simulink model "SecRwLtStLgrstInwdOtwdIsPosChk"  (R2024b)
settings: Solver=FixedStepDiscrete  StartTime=0.0  StopTime=10.0  FixedStep=0.01  RelTol=1e-3
undefined symbols (not defined in the file or in its folder): KeSMSuSecRwStLegrestInOutPosDelta_Val, KeSMSuSecRwStLegrestInOutPosTolr_Val
libraries: StIsPosChkLib x12, simulink x7
(part 1 of 2)
settings Model: Creator=sn2xws  LastModifiedBy=sn55gm
settings Model: ModifiedHistory=|
  | 2023.8.1 V2.0.0 CR421790 增加模式21-26
  | 2023.9.14 V2.1.0 Bug 540886 修改模式判断到位的条件为10ms周期计算
  | 2024.5.8 V3.0.0 557 eze 模式变更
  | 2024.8.15 V3.0.1 智享模式需要计算目标位置，不能直接判断到位置，posalready赋值0
  | 2024.9.5 V3.0.2 增加Md56，注释不用的模式
  | 2024.12.17 V3.0.3 Md57 Md58 报失败问题
  | 25.7.1 V3.13.0 新增MD61 MD62
  | 2510.10V3.13.2 二排腿托都动完再停发目标位置
settings SolverCC: AlgebraicLoopSolver=TrustRegion
settings DataIOCC: SaveFormat=StructureWithTime  ReturnWorkspaceOutputs=off
settings OptimizationCC: DefaultParameterBehavior=Inlined  EnhancedBackFolding=on  PassReuseOutputArgsAs=Individual arguments  ZeroExternalMemoryAtStartup=off  ZeroInternalMemoryAtStartup=off  OptimizeBlockOrder=speed  DifferentSizesBufferReuse=on  OptimizationCustomize=off  EfficientTunableParamExpr=on
settings DebuggingCC: ParameterTunabilityLossMsg=error  UnconnectedInputMsg=warning  UnconnectedOutputMsg=warning  UnconnectedLineMsg=warning  ArithmeticOperatorsInVariantConditions=warning
settings ModelReferenceCC: EnableRefExpFcnMdlSchedulingChecks=on  ModelReferenceNumInstancesAllowed=Single
settings SFSimCC: MATLABDynamicMemAlloc=off  CustomCodeUndefinedFunction=UseInterfaceOnly
settings RTWCC: Description=AUTOSAR  SystemTargetFile=autosar.tlc  GenCodeOnly=on  TemplateMakefile=ert_default_tmf  GenerateReport=on  IncludeHyperlinkInReport=on  LaunchReport=on  DataTypeReplacement=CDataTypesFixedWidth  GenerateTraceInfo=on  GenerateTraceReport=on  GenerateTraceReportSl=on  GenerateTraceReportSf=on  GenerateTraceReportEml=on  GenerateCodeMetricsReport=on  GPUComputeCapability=3.5
settings CodeAppCC: ForceParamTrailComments=on  IgnoreCustomStorageClasses=off  OperatorAnnotations=on  SimulinkDataObjDesc=on  SFDataObjDesc=on  InsertBlockDesc=on
settings STFCustomTargetCC: TargetLangStandard=C99 (ISO)  MultiwordLength=256  ParMdlRefBuildCompliant=on  CompOptLevelCompliant=on  IncludeMdlTerminateFcn=off  CombineOutputUpdateFcns=on  SuppressErrorStatus=on  ERTCustomFileBanners=on  SupportNonFinite=off  SupportComplex=off  SupportContinuousTime=off  SupportNonInlinedSFcns=off  RemoveResetFunc=on  MATLABClassNameForMDSCustomization=Simulink.SoftwareTarget.ERTCustomization  AutosarCompliant=on  UseToolchainInfoCompliant=on  LookupTableObjectStructAxisOrder=2,1,3,4,...  LUTObjectStructOrderEvenSpacing=Size,Table,Breakpoints  SystemTargetFile=autosar.tlc
settings ERTTargetCC: TargetLangStandard=C99 (ISO)  ConcurrentExecutionCompliant=off  IncludeMdlTerminateFcn=off  SuppressErrorStatus=on  SupportNonFinite=off  SupportComplex=off  ModelStepFunctionPrototypeControlCompliant=off  CPPClassGenCompliant=off  AutosarCompliant=on  LookupTableObjectStructAxisOrder=2,1,3,4,...  LUTObjectStructOrderEvenSpacing=Size,Table,Breakpoints  ERTCustomFileTemplate=example_file_process.tlc  ERTFilePackagingFormat=Compact  BooleanTrueId=TRUE  BooleanFalseId=FALSE  DynamicArrayContainerType=coder::array

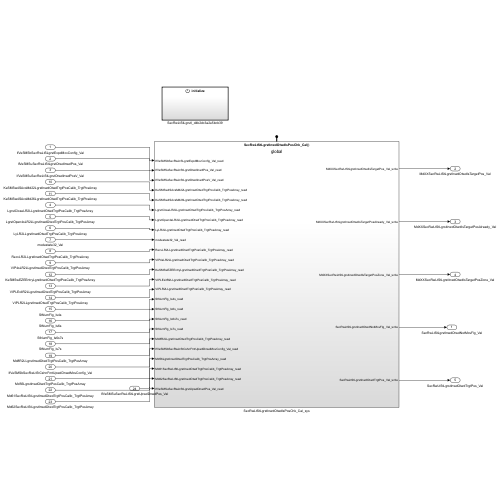
[thumbnail: Simulink's stored preview of the top-level diagram]
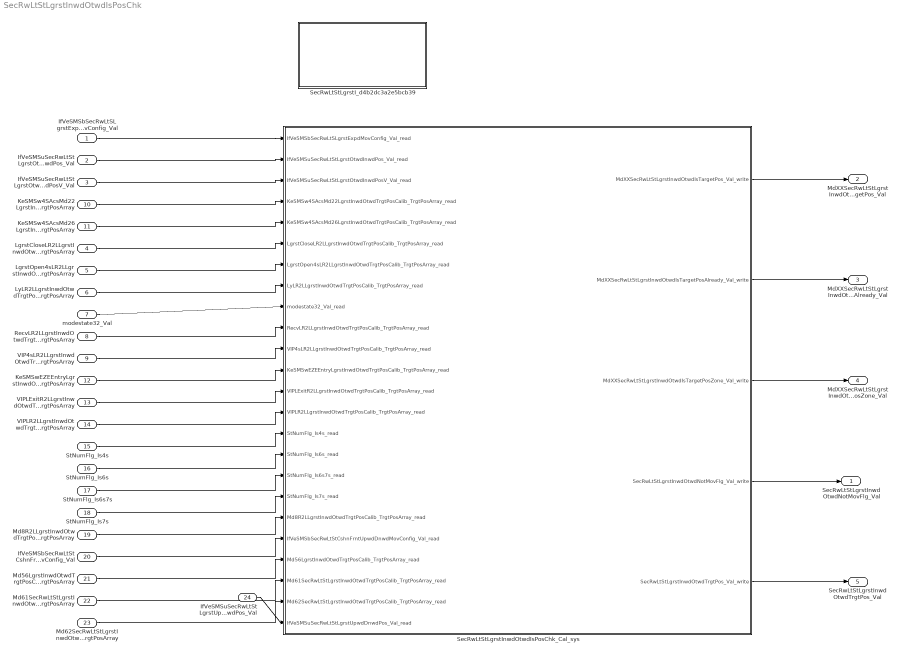
== system SecRwLtStLgrstInwdOtwdIsPosChk ==
  IfVeSMSbSecRwLtSLgrstExpdMovConfig_Val : Inport  OutDataTypeStr=boolean  PortDimensions=1
  IfVeSMSuSecRwLtStLgrstOtwdInwdPos_Val : Inport  Port=2  OutDataTypeStr=uint16  PortDimensions=1
  IfVeSMSuSecRwLtStLgrstOtwdInwdPosV_Val : Inport  Port=3  OutDataTypeStr=boolean  PortDimensions=1
  LgrstCloseLR2LLgrstInwdOtwdTrgtPosCalib_TrgtPosArray : Inport  Description=|  Port=4  OutDataTypeStr=uint16  PortDimensions=3
      | 0:Pos
      | 1:Max
      | 2:Min
  LgrstOpen4sLR2LLgrstInwdOtwdTrgtPosCalib_TrgtPosArray : Inport  Description=|  Port=5  OutDataTypeStr=uint16  PortDimensions=3
      | 0:Pos
      | 1:Max
      | 2:Min
  LyLR2LLgrstInwdOtwdTrgtPosCalib_TrgtPosArray : Inport  Description=|  Port=6  OutDataTypeStr=uint16  PortDimensions=3
      | 0:Pos
      | 1:Max
      | 2:Min
  modestate32_Val : Inport  Port=7  OutDataTypeStr=uint32  PortDimensions=1
  RecvLR2LLgrstInwdOtwdTrgtPosCalib_TrgtPosArray : Inport  Description=|  Port=8  OutDataTypeStr=uint16  PortDimensions=3
      | 0:Pos
      | 1:Max
      | 2:Min
  VIP4sLR2LLgrstInwdOtwdTrgtPosCalib_TrgtPosArray : Inport  Description=|  Port=9  OutDataTypeStr=uint16  PortDimensions=3
      | 0:Pos
      | 1:Max
      | 2:Min
  KeSMSw4SAcsMd22LgrstInwdOtwdTrgtPosCalib_TrgtPosArray : Inport  Description=|  Port=10  OutDataTypeStr=uint16  PortDimensions=3
      | 0:Pos
      | 1:Max
      | 2:Min
  KeSMSw4SAcsMd26LgrstInwdOtwdTrgtPosCalib_TrgtPosArray : Inport  Description=|  Port=11  OutDataTypeStr=uint16  PortDimensions=3
      | 0:Pos
      | 1:Max
      | 2:Min
  KeSMSwEZEEntryLgrstInwdOtwdTrgtPosCalib_TrgtPosArray : Inport  Description=|  Port=12  OutDataTypeStr=uint16  PortDimensions=3
      | 0:Pos
      | 1:Max
      | 2:Min
  VIPLExitR2LLgrstInwdOtwdTrgtPosCalib_TrgtPosArray : Inport  Description=|  Port=13  OutDataTypeStr=uint16  PortDimensions=3
      | 0:Pos
      | 1:Max
      | 2:Min
  VIPLR2LLgrstInwdOtwdTrgtPosCalib_TrgtPosArray : Inport  Description=|  Port=14  OutDataTypeStr=uint16  PortDimensions=3
      | 0:Pos
      | 1:Max
      | 2:Min
  StNumFlg_Is4s : Inport  Port=15  OutDataTypeStr=boolean  PortDimensions=1
  StNumFlg_Is6s : Inport  Port=16  OutDataTypeStr=boolean  PortDimensions=1
  StNumFlg_Is6s7s : Inport  Port=17  OutDataTypeStr=boolean  PortDimensions=1
  StNumFlg_Is7s : Inport  Port=18  OutDataTypeStr=boolean  PortDimensions=1
  Md8R2LLgrstInwdOtwdTrgtPosCalib_TrgtPosArray : Inport  Description=|  Port=19  OutDataTypeStr=uint16  PortDimensions=3
      | 0:Pos
      | 1:Max
      | 2:Min
  IfVeSMSbSecRwLtStCshnFrntUpwdDnwdMovConfig_Val : Inport  Port=20  OutDataTypeStr=boolean  PortDimensions=1
  Md56LgrstInwdOtwdTrgtPosCalib_TrgtPosArray : Inport  Description=|  Port=21  OutDataTypeStr=uint16  PortDimensions=3
      | 0:Pos
      | 1:Max
      | 2:Min
  Md61SecRwLtStLgrstInwdOtwdTrgtPosCalib_TrgtPosArray : Inport  Description=|  Port=22  OutDataTypeStr=uint16  PortDimensions=3
      | 0:Pos
      | 1:Max
      | 2:Min
  Md62SecRwLtStLgrstInwdOtwdTrgtPosCalib_TrgtPosArray : Inport  Description=|  Port=23  OutDataTypeStr=uint16  PortDimensions=3
      | 0:Pos
      | 1:Max
      | 2:Min
  IfVeSMSuSecRwLtStLgrstUpwdDnwdPos_Val : Inport  Port=24  OutDataTypeStr=uint16  PortDimensions=1
  SecRwLtStLgrstI_d4b2dc3a2e5bcb39 : Subsystem
  SecRwLtStLgrstInwdOtwdIsPosChk_Cal_sys : Subsystem
  SecRwLtStLgrstInwdOtwdNotMovFlg_Val : Outport  OutDataTypeStr=boolean  PortDimensions=1  VectorParamsAs1DForOutWhenUnconnected=off
  MdXXSecRwLtStLgrstInwdOtwdIsTargetPos_Val : Outport  Port=2  OutDataTypeStr=uint32  PortDimensions=1  VectorParamsAs1DForOutWhenUnconnected=off
  MdXXSecRwLtStLgrstInwdOtwdIsTargetPosAlready_Val : Outport  Port=3  OutDataTypeStr=uint32  PortDimensions=1  VectorParamsAs1DForOutWhenUnconnected=off
  MdXXSecRwLtStLgrstInwdOtwdIsTargetPosZone_Val : Outport  Port=4  OutDataTypeStr=uint32  PortDimensions=1  VectorParamsAs1DForOutWhenUnconnected=off
  SecRwLtStLgrstInwdOtwdTrgtPos_Val : Outport  Port=5  OutDataTypeStr=uint16  PortDimensions=1  VectorParamsAs1DForOutWhenUnconnected=off
  wires:
  IfVeSMSbSecRwLtSLgrstExpdMovConfig_Val/1 -> SecRwLtStLgrstInwdOtwdIsPosChk_Cal_sys/1(IfVeSMSbSecRwLtSLgrstExpdMovConfig_Val_read)
  IfVeSMSuSecRwLtStLgrstOtwdInwdPos_Val/1 -> SecRwLtStLgrstInwdOtwdIsPosChk_Cal_sys/2(IfVeSMSuSecRwLtStLgrstOtwdInwdPos_Val_read)
  IfVeSMSuSecRwLtStLgrstOtwdInwdPosV_Val/1 -> SecRwLtStLgrstInwdOtwdIsPosChk_Cal_sys/3(IfVeSMSuSecRwLtStLgrstOtwdInwdPosV_Val_read)
  LgrstCloseLR2LLgrstInwdOtwdTrgtPosCalib_TrgtPosArray/1 -> SecRwLtStLgrstInwdOtwdIsPosChk_Cal_sys/6(LgrstCloseLR2LLgrstInwdOtwdTrgtPosCalib_TrgtPosArray_read)
  LgrstOpen4sLR2LLgrstInwdOtwdTrgtPosCalib_TrgtPosArray/1 -> SecRwLtStLgrstInwdOtwdIsPosChk_Cal_sys/7(LgrstOpen4sLR2LLgrstInwdOtwdTrgtPosCalib_TrgtPosArray_read)
  LyLR2LLgrstInwdOtwdTrgtPosCalib_TrgtPosArray/1 -> SecRwLtStLgrstInwdOtwdIsPosChk_Cal_sys/8(LyLR2LLgrstInwdOtwdTrgtPosCalib_TrgtPosArray_read)
  modestate32_Val/1 -> SecRwLtStLgrstInwdOtwdIsPosChk_Cal_sys/9(modestate32_Val_read)
  RecvLR2LLgrstInwdOtwdTrgtPosCalib_TrgtPosArray/1 -> SecRwLtStLgrstInwdOtwdIsPosChk_Cal_sys/10(RecvLR2LLgrstInwdOtwdTrgtPosCalib_TrgtPosArray_read)
  VIP4sLR2LLgrstInwdOtwdTrgtPosCalib_TrgtPosArray/1 -> SecRwLtStLgrstInwdOtwdIsPosChk_Cal_sys/11(VIP4sLR2LLgrstInwdOtwdTrgtPosCalib_TrgtPosArray_read)
  SecRwLtStLgrstInwdOtwdIsPosChk_Cal_sys/1(MdXXSecRwLtStLgrstInwdOtwdIsTargetPos_Val_write) -> MdXXSecRwLtStLgrstInwdOtwdIsTargetPos_Val/1
  SecRwLtStLgrstInwdOtwdIsPosChk_Cal_sys/2(MdXXSecRwLtStLgrstInwdOtwdIsTargetPosAlready_Val_write) -> MdXXSecRwLtStLgrstInwdOtwdIsTargetPosAlready_Val/1
  SecRwLtStLgrstInwdOtwdIsPosChk_Cal_sys/3(MdXXSecRwLtStLgrstInwdOtwdIsTargetPosZone_Val_write) -> MdXXSecRwLtStLgrstInwdOtwdIsTargetPosZone_Val/1
  SecRwLtStLgrstInwdOtwdIsPosChk_Cal_sys/4(SecRwLtStLgrstInwdOtwdNotMovFlg_Val_write) -> SecRwLtStLgrstInwdOtwdNotMovFlg_Val/1
  SecRwLtStLgrstInwdOtwdIsPosChk_Cal_sys/5(SecRwLtStLgrstInwdOtwdTrgtPos_Val_write) -> SecRwLtStLgrstInwdOtwdTrgtPos_Val/1
  KeSMSw4SAcsMd22LgrstInwdOtwdTrgtPosCalib_TrgtPosArray/1 -> SecRwLtStLgrstInwdOtwdIsPosChk_Cal_sys/4(KeSMSw4SAcsMd22LgrstInwdOtwdTrgtPosCalib_TrgtPosArray_read)
  KeSMSw4SAcsMd26LgrstInwdOtwdTrgtPosCalib_TrgtPosArray/1 -> SecRwLtStLgrstInwdOtwdIsPosChk_Cal_sys/5(KeSMSw4SAcsMd26LgrstInwdOtwdTrgtPosCalib_TrgtPosArray_read)
  KeSMSwEZEEntryLgrstInwdOtwdTrgtPosCalib_TrgtPosArray/1 -> SecRwLtStLgrstInwdOtwdIsPosChk_Cal_sys/12(KeSMSwEZEEntryLgrstInwdOtwdTrgtPosCalib_TrgtPosArray_read)
  VIPLExitR2LLgrstInwdOtwdTrgtPosCalib_TrgtPosArray/1 -> SecRwLtStLgrstInwdOtwdIsPosChk_Cal_sys/13(VIPLExitR2LLgrstInwdOtwdTrgtPosCalib_TrgtPosArray_read)
  VIPLR2LLgrstInwdOtwdTrgtPosCalib_TrgtPosArray/1 -> SecRwLtStLgrstInwdOtwdIsPosChk_Cal_sys/14(VIPLR2LLgrstInwdOtwdTrgtPosCalib_TrgtPosArray_read)
  StNumFlg_Is4s/1 -> SecRwLtStLgrstInwdOtwdIsPosChk_Cal_sys/15(StNumFlg_Is4s_read)
  StNumFlg_Is6s/1 -> SecRwLtStLgrstInwdOtwdIsPosChk_Cal_sys/16(StNumFlg_Is6s_read)
  StNumFlg_Is6s7s/1 -> SecRwLtStLgrstInwdOtwdIsPosChk_Cal_sys/17(StNumFlg_Is6s7s_read)
  StNumFlg_Is7s/1 -> SecRwLtStLgrstInwdOtwdIsPosChk_Cal_sys/18(StNumFlg_Is7s_read)
  Md8R2LLgrstInwdOtwdTrgtPosCalib_TrgtPosArray/1 -> SecRwLtStLgrstInwdOtwdIsPosChk_Cal_sys/19(Md8R2LLgrstInwdOtwdTrgtPosCalib_TrgtPosArray_read)
  IfVeSMSbSecRwLtStCshnFrntUpwdDnwdMovConfig_Val/1 -> SecRwLtStLgrstInwdOtwdIsPosChk_Cal_sys/20(IfVeSMSbSecRwLtStCshnFrntUpwdDnwdMovConfig_Val_read)
  Md56LgrstInwdOtwdTrgtPosCalib_TrgtPosArray/1 -> SecRwLtStLgrstInwdOtwdIsPosChk_Cal_sys/21(Md56LgrstInwdOtwdTrgtPosCalib_TrgtPosArray_read)
  Md61SecRwLtStLgrstInwdOtwdTrgtPosCalib_TrgtPosArray/1 -> SecRwLtStLgrstInwdOtwdIsPosChk_Cal_sys/22(Md61SecRwLtStLgrstInwdOtwdTrgtPosCalib_TrgtPosArray_read)
  Md62SecRwLtStLgrstInwdOtwdTrgtPosCalib_TrgtPosArray/1 -> SecRwLtStLgrstInwdOtwdIsPosChk_Cal_sys/23(Md62SecRwLtStLgrstInwdOtwdTrgtPosCalib_TrgtPosArray_read)
  IfVeSMSuSecRwLtStLgrstUpwdDnwdPos_Val/1 -> SecRwLtStLgrstInwdOtwdIsPosChk_Cal_sys/24(IfVeSMSuSecRwLtStLgrstUpwdDnwdPos_Val_read)

== system SecRwLtStLgrstInwdOtwdIsPosChk/SecRwLtStLgrstI_d4b2dc3a2e5bcb39 ==
  note: Added blocks
  note: Added blocks
  Event Listener : EventListener  EventName=reset
  PA_KeSMSuSecRwStLegrestInOutPosDelta_Val : Constant  Value=KeSMSuSecRwStLegrestInOutPosDelta_Val
  PA_KeSMSuSecRwStLegrestInOutPosTolr_Val : Constant  Value=KeSMSuSecRwStLegrestInOutPosTolr_Val
  Terminator_1 : Terminator
  Terminator_2 : Terminator
  wires:
  PA_KeSMSuSecRwStLegrestInOutPosDelta_Val/1 -> Terminator_1/1
  PA_KeSMSuSecRwStLegrestInOutPosTolr_Val/1 -> Terminator_2/1

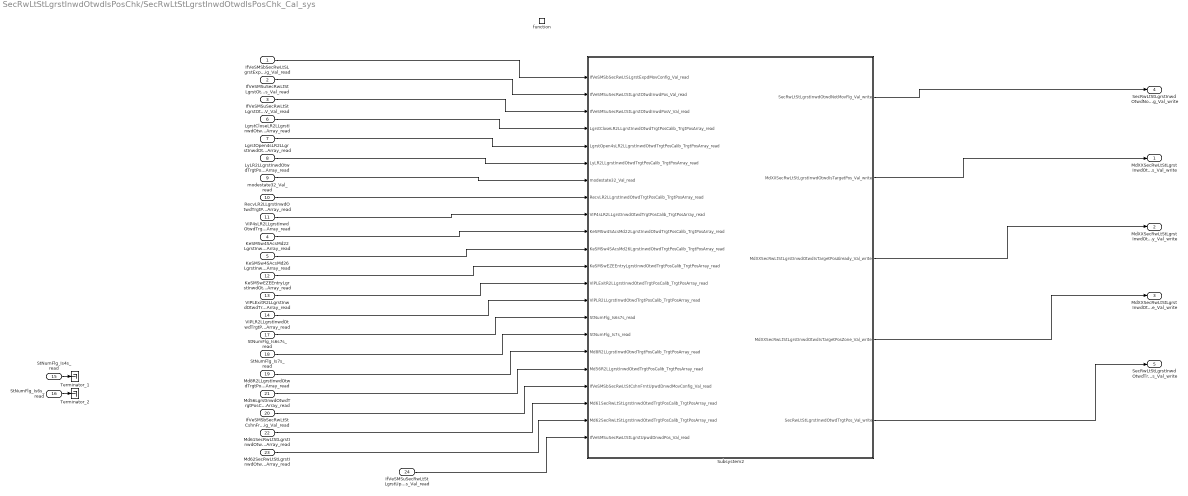
== system SecRwLtStLgrstInwdOtwdIsPosChk/SecRwLtStLgrstInwdOtwdIsPosChk_Cal_sys ==
  IfVeSMSbSecRwLtSLgrstExpdMovConfig_Val_read : Inport
  IfVeSMSuSecRwLtStLgrstOtwdInwdPos_Val_read : Inport  Port=2
  IfVeSMSuSecRwLtStLgrstOtwdInwdPosV_Val_read : Inport  Port=3
  KeSMSw4SAcsMd22LgrstInwdOtwdTrgtPosCalib_TrgtPosArray_read : Inport  Port=4
  KeSMSw4SAcsMd26LgrstInwdOtwdTrgtPosCalib_TrgtPosArray_read : Inport  Port=5
  LgrstCloseLR2LLgrstInwdOtwdTrgtPosCalib_TrgtPosArray_read : Inport  Port=6
  LgrstOpen4sLR2LLgrstInwdOtwdTrgtPosCalib_TrgtPosArray_read : Inport  Port=7
  LyLR2LLgrstInwdOtwdTrgtPosCalib_TrgtPosArray_read : Inport  Port=8
  modestate32_Val_read : Inport  Port=9
  RecvLR2LLgrstInwdOtwdTrgtPosCalib_TrgtPosArray_read : Inport  Port=10
  VIP4sLR2LLgrstInwdOtwdTrgtPosCalib_TrgtPosArray_read : Inport  Port=11
  KeSMSwEZEEntryLgrstInwdOtwdTrgtPosCalib_TrgtPosArray_read : Inport  Port=12
  VIPLExitR2LLgrstInwdOtwdTrgtPosCalib_TrgtPosArray_read : Inport  Port=13
  VIPLR2LLgrstInwdOtwdTrgtPosCalib_TrgtPosArray_read : Inport  Port=14
  StNumFlg_Is4s_read : Inport  Port=15
  StNumFlg_Is6s_read : Inport  Port=16
  StNumFlg_Is6s7s_read : Inport  Port=17
  StNumFlg_Is7s_read : Inport  Port=18
  Md8R2LLgrstInwdOtwdTrgtPosCalib_TrgtPosArray_read : Inport  Port=19
  IfVeSMSbSecRwLtStCshnFrntUpwdDnwdMovConfig_Val_read : Inport  Port=20
  Md56LgrstInwdOtwdTrgtPosCalib_TrgtPosArray_read : Inport  Port=21
  Md61SecRwLtStLgrstInwdOtwdTrgtPosCalib_TrgtPosArray_read : Inport  Port=22
  Md62SecRwLtStLgrstInwdOtwdTrgtPosCalib_TrgtPosArray_read : Inport  Port=23
  IfVeSMSuSecRwLtStLgrstUpwdDnwdPos_Val_read : Inport  Port=24
  function : TriggerPort  TriggerType=function-call  IsSimulinkFunction=on  FunctionName=SecRwLtStLgrstInwdOtwdIsPosChk_Cal  VariantControl=(inherit)
  Subsystem2 : Subsystem
  Terminator_1 : Terminator
  Terminator_2 : Terminator
  MdXXSecRwLtStLgrstInwdOtwdIsTargetPos_Val_write : Outport  VectorParamsAs1DForOutWhenUnconnected=off
      settings: EnsureOutportIsVirtual=on
  MdXXSecRwLtStLgrstInwdOtwdIsTargetPosAlready_Val_write : Outport  Port=2  VectorParamsAs1DForOutWhenUnconnected=off
      settings: EnsureOutportIsVirtual=on
  MdXXSecRwLtStLgrstInwdOtwdIsTargetPosZone_Val_write : Outport  Port=3  VectorParamsAs1DForOutWhenUnconnected=off
      settings: EnsureOutportIsVirtual=on
  SecRwLtStLgrstInwdOtwdNotMovFlg_Val_write : Outport  Port=4  VectorParamsAs1DForOutWhenUnconnected=off
      settings: EnsureOutportIsVirtual=on
  SecRwLtStLgrstInwdOtwdTrgtPos_Val_write : Outport  Port=5  VectorParamsAs1DForOutWhenUnconnected=off
      settings: EnsureOutportIsVirtual=on
  wires:
  LgrstCloseLR2LLgrstInwdOtwdTrgtPosCalib_TrgtPosArray_read/1 -> Subsystem2/4(LgrstCloseLR2LLgrstInwdOtwdTrgtPosCalib_TrgtPosArray_read)
  IfVeSMSuSecRwLtStLgrstOtwdInwdPos_Val_read/1 -> Subsystem2/2(IfVeSMSuSecRwLtStLgrstOtwdInwdPos_Val_read)
  IfVeSMSuSecRwLtStLgrstOtwdInwdPosV_Val_read/1 -> Subsystem2/3(IfVeSMSuSecRwLtStLgrstOtwdInwdPosV_Val_read)
  LgrstOpen4sLR2LLgrstInwdOtwdTrgtPosCalib_TrgtPosArray_read/1 -> Subsystem2/5(LgrstOpen4sLR2LLgrstInwdOtwdTrgtPosCalib_TrgtPosArray_read)
  IfVeSMSbSecRwLtSLgrstExpdMovConfig_Val_read/1 -> Subsystem2/1(IfVeSMSbSecRwLtSLgrstExpdMovConfig_Val_read)
  LyLR2LLgrstInwdOtwdTrgtPosCalib_TrgtPosArray_read/1 -> Subsystem2/6(LyLR2LLgrstInwdOtwdTrgtPosCalib_TrgtPosArray_read)
  modestate32_Val_read/1 -> Subsystem2/7(modestate32_Val_read)
  RecvLR2LLgrstInwdOtwdTrgtPosCalib_TrgtPosArray_read/1 -> Subsystem2/8(RecvLR2LLgrstInwdOtwdTrgtPosCalib_TrgtPosArray_read)
  VIP4sLR2LLgrstInwdOtwdTrgtPosCalib_TrgtPosArray_read/1 -> Subsystem2/9(VIP4sLR2LLgrstInwdOtwdTrgtPosCalib_TrgtPosArray_read)
  KeSMSw4SAcsMd22LgrstInwdOtwdTrgtPosCalib_TrgtPosArray_read/1 -> Subsystem2/10(KeSMSw4SAcsMd22LgrstInwdOtwdTrgtPosCalib_TrgtPosArray_read)
  KeSMSw4SAcsMd26LgrstInwdOtwdTrgtPosCalib_TrgtPosArray_read/1 -> Subsystem2/11(KeSMSw4SAcsMd26LgrstInwdOtwdTrgtPosCalib_TrgtPosArray_read)
  Subsystem2/1(SecRwLtStLgrstInwdOtwdNotMovFlg_Val_write) -> SecRwLtStLgrstInwdOtwdNotMovFlg_Val_write/1
  Subsystem2/2(MdXXSecRwLtStLgrstInwdOtwdIsTargetPos_Val_write) -> MdXXSecRwLtStLgrstInwdOtwdIsTargetPos_Val_write/1
  Subsystem2/3(MdXXSecRwLtStLgrstInwdOtwdIsTargetPosAlready_Val_write) -> MdXXSecRwLtStLgrstInwdOtwdIsTargetPosAlready_Val_write/1
  Subsystem2/4(MdXXSecRwLtStLgrstInwdOtwdIsTargetPosZone_Val_write) -> MdXXSecRwLtStLgrstInwdOtwdIsTargetPosZone_Val_write/1
  Subsystem2/5(SecRwLtStLgrstInwdOtwdTrgtPos_Val_write) -> SecRwLtStLgrstInwdOtwdTrgtPos_Val_write/1
  KeSMSwEZEEntryLgrstInwdOtwdTrgtPosCalib_TrgtPosArray_read/1 -> Subsystem2/12(KeSMSwEZEEntryLgrstInwdOtwdTrgtPosCalib_TrgtPosArray_read)
  VIPLExitR2LLgrstInwdOtwdTrgtPosCalib_TrgtPosArray_read/1 -> Subsystem2/13(VIPLExitR2LLgrstInwdOtwdTrgtPosCalib_TrgtPosArray_read)
  VIPLR2LLgrstInwdOtwdTrgtPosCalib_TrgtPosArray_read/1 -> Subsystem2/14(VIPLR2LLgrstInwdOtwdTrgtPosCalib_TrgtPosArray_read)
  StNumFlg_Is4s_read/1 -> Terminator_1/1
  StNumFlg_Is6s_read/1 -> Terminator_2/1
  StNumFlg_Is6s7s_read/1 -> Subsystem2/15(StNumFlg_Is6s7s_read)
  StNumFlg_Is7s_read/1 -> Subsystem2/16(StNumFlg_Is7s_read)
  Md8R2LLgrstInwdOtwdTrgtPosCalib_TrgtPosArray_read/1 -> Subsystem2/17(Md8R2LLgrstInwdOtwdTrgtPosCalib_TrgtPosArray_read)
  Md56LgrstInwdOtwdTrgtPosCalib_TrgtPosArray_read/1 -> Subsystem2/18(Md56R2LLgrstInwdOtwdTrgtPosCalib_TrgtPosArray_read)
  IfVeSMSbSecRwLtStCshnFrntUpwdDnwdMovConfig_Val_read/1 -> Subsystem2/19(IfVeSMSbSecRwLtStCshnFrntUpwdDnwdMovConfig_Val_read)
  Md61SecRwLtStLgrstInwdOtwdTrgtPosCalib_TrgtPosArray_read/1 -> Subsystem2/20(Md61SecRwLtStLgrstInwdOtwdTrgtPosCalib_TrgtPosArray_read)
  Md62SecRwLtStLgrstInwdOtwdTrgtPosCalib_TrgtPosArray_read/1 -> Subsystem2/21(Md62SecRwLtStLgrstInwdOtwdTrgtPosCalib_TrgtPosArray_read)
  IfVeSMSuSecRwLtStLgrstUpwdDnwdPos_Val_read/1 -> Subsystem2/22(IfVeSMSuSecRwLtStLgrstUpwdDnwdPos_Val_read)

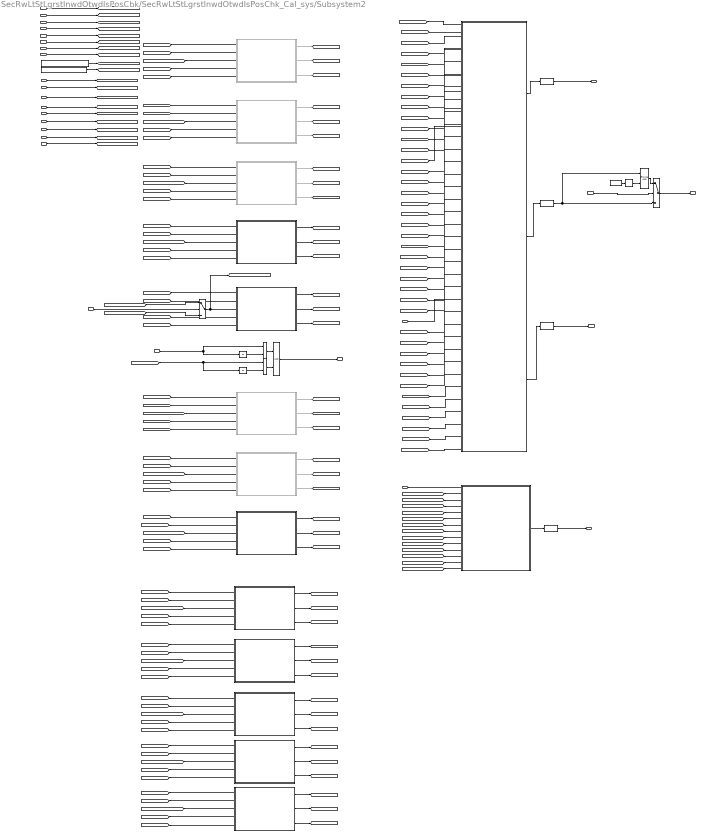
== system SecRwLtStLgrstInwdOtwdIsPosChk/SecRwLtStLgrstInwdOtwdIsPosChk_Cal_sys/Subsystem2 ==
  note: 2023.9.14 V2.1.0 Bug 540886 修改模式判断到位的条件为10ms周期计算
  note: 2023.8.1 V2.0.0 CR421790 增加模式21-26
  IfVeSMSbSecRwLtSLgrstExpdMovConfig_Val_read : Inport
  IfVeSMSuSecRwLtStLgrstOtwdInwdPos_Val_read : Inport  Port=2
  IfVeSMSuSecRwLtStLgrstOtwdInwdPosV_Val_read : Inport  Port=3
  LgrstCloseLR2LLgrstInwdOtwdTrgtPosCalib_TrgtPosArray_read : Inport  Port=4
  LgrstOpen4sLR2LLgrstInwdOtwdTrgtPosCalib_TrgtPosArray_read : Inport  Port=5
  LyLR2LLgrstInwdOtwdTrgtPosCalib_TrgtPosArray_read : Inport  Port=6
  modestate32_Val_read : Inport  Port=7
  RecvLR2LLgrstInwdOtwdTrgtPosCalib_TrgtPosArray_read : Inport  Port=8
  VIP4sLR2LLgrstInwdOtwdTrgtPosCalib_TrgtPosArray_read : Inport  Port=9
  KeSMSw4SAcsMd22LgrstInwdOtwdTrgtPosCalib_TrgtPosArray_read : Inport  Port=10
  KeSMSw4SAcsMd26LgrstInwdOtwdTrgtPosCalib_TrgtPosArray_read : Inport  Port=11
  KeSMSwEZEEntryLgrstInwdOtwdTrgtPosCalib_TrgtPosArray_read : Inport  Port=12
  VIPLExitR2LLgrstInwdOtwdTrgtPosCalib_TrgtPosArray_read : Inport  Port=13
  VIPLR2LLgrstInwdOtwdTrgtPosCalib_TrgtPosArray_read : Inport  Port=14
  StNumFlg_Is6s7s_read : Inport  Port=15
  StNumFlg_Is7s_read : Inport  Port=16
  Md8R2LLgrstInwdOtwdTrgtPosCalib_TrgtPosArray_read : Inport  Port=17
  Md56R2LLgrstInwdOtwdTrgtPosCalib_TrgtPosArray_read : Inport  Port=18
  IfVeSMSbSecRwLtStCshnFrntUpwdDnwdMovConfig_Val_read : Inport  Port=19
  Md61SecRwLtStLgrstInwdOtwdTrgtPosCalib_TrgtPosArray_read : Inport  Port=20
  Md62SecRwLtStLgrstInwdOtwdTrgtPosCalib_TrgtPosArray_read : Inport  Port=21
  IfVeSMSuSecRwLtStLgrstUpwdDnwdPos_Val_read : Inport  Port=22
  Bitwise Operator : simulink/Logic and Bit Operations/Bitwise Operator  logicop=AND  UseBitMask=off  NumInputPorts=2  BitMask=bin2dec('11011001')  BitMaskRealWorld=Stored Integer
  Bitwise Operator1 : simulink/Logic and Bit Operations/Bitwise Operator  logicop=NOT  UseBitMask=off  BitMask=bin2dec('11011001')  BitMaskRealWorld=Stored Integer
  Constant : Constant  Value=512  OutDataTypeStr=uint32
  Data Type Conversion{,1..3} (4 alike) : DataTypeConversion  SaturateOnIntegerOverflow=off  RndMeth=Floor
  Logical Operator3 : Logic  AllPortsSameDT=off  OutDataTypeStr=boolean
  PA_KeSMSuSecRwStLegrestInOutPosDelta_Val : Constant  Value=KeSMSuSecRwStLegrestInOutPosDelta_Val
  PA_KeSMSuSecRwStLegrestInOutPosTolr_Val : Constant  Value=KeSMSuSecRwStLegrestInOutPosTolr_Val
  Relational Operator2 : RelationalOperator  Operator===  OutDataTypeStr=boolean  RndMeth=Simplest  InputSameDT=off
  Relational Operator3 : RelationalOperator  Operator===  OutDataTypeStr=boolean  RndMeth=Simplest  InputSameDT=off
  Subsystem : Subsystem
  Subsystem1 : Subsystem
  Subsystem10 : Subsystem
  Subsystem11 : Subsystem
  Subsystem12 : Subsystem
  Subsystem13 : Subsystem
  Subsystem14 : Subsystem
  Subsystem2 : Subsystem  Commented=on
  Subsystem3 : Subsystem  Commented=on
  Subsystem4 : Subsystem  Commented=on
  Subsystem5 : Subsystem
  Subsystem6 : Subsystem
  Subsystem7 : Subsystem  Commented=on
  Subsystem8 : Subsystem  Commented=on
  Subsystem9 : Subsystem
  Switch : Switch  Criteria=u2 > Threshold  SaturateOnIntegerOverflow=off  InputSameDT=off
  Switch1 : Switch  Criteria=u2 > Threshold  SaturateOnIntegerOverflow=off  InputSameDT=off
  Unit Delay2 : UnitDelay  SampleTime=-1  HasFrameUpgradeWarning=on
  Unit Delay3 : UnitDelay  SampleTime=-1  HasFrameUpgradeWarning=on
  SecRwLtStLgrstInwdOtwdNotMovFlg_Val_write : Outport  VectorParamsAs1DForOutWhenUnconnected=off
      settings: EnsureOutportIsVirtual=on
  MdXXSecRwLtStLgrstInwdOtwdIsTargetPos_Val_write : Outport  Port=2  VectorParamsAs1DForOutWhenUnconnected=off
      settings: EnsureOutportIsVirtual=on
  MdXXSecRwLtStLgrstInwdOtwdIsTargetPosAlready_Val_write : Outport  Port=3  VectorParamsAs1DForOutWhenUnconnected=off
      settings: EnsureOutportIsVirtual=on
  MdXXSecRwLtStLgrstInwdOtwdIsTargetPosZone_Val_write : Outport  Port=4  VectorParamsAs1DForOutWhenUnconnected=off
      settings: EnsureOutportIsVirtual=on
  SecRwLtStLgrstInwdOtwdTrgtPos_Val_write : Outport  Port=5  VectorParamsAs1DForOutWhenUnconnected=off
      settings: EnsureOutportIsVirtual=on
  wires:
  [PosTolr] -> Subsystem5/5(Tolr)
  PA_KeSMSuSecRwStLegrestInOutPosTolr_Val/1 -> [PosTolr]
  [PosTolr] -> Subsystem6/5(Tolr)
  LgrstCloseLR2LLgrstInwdOtwdTrgtPosCalib_TrgtPosArray_read/1 -> [LgrstCloseLCalib]
  Subsystem1/3(IsTargetPosZone) -> Data Type Conversion3/1
  [PosTolr] -> Subsystem4/5(Tolr)
  [LgrstOpenLIsTargetPosAlready] -> ?
  [LgrstOpenLCalib] -> Subsystem/2(LgrstOpenLCalib)
  [PosTolr] -> Subsystem3/5(Tolr)
  Subsystem1/1(IsTargetPos) -> Data Type Conversion1/1
  IfVeSMSuSecRwLtStLgrstOtwdInwdPosV_Val_read/1 -> [PosV]
  [LgrstOpenLIsTargetPos] -> ?
  VIP4sLR2LLgrstInwdOtwdTrgtPosCalib_TrgtPosArray_read/1 -> [VIPL4sCalib]
  Subsystem4/2(IsPosZone) -> [LyLIsTargetPosZone]
  [VIPLIsTargetPosAlready] -> Subsystem1/7(VIPLIsTargetPosAlready)
  [VIPLCalib] -> Subsystem/6(VIPLCalib)
  [PosDelta] -> Subsystem3/4(Delta)
  [Pos] -> Subsystem3/2(Pos)
  Subsystem2/2(IsPosZone) -> [LgrstOpenLIsTargetPosZone]
  IfVeSMSbSecRwLtSLgrstExpdMovConfig_Val_read/1 -> [MovConfig]
  PA_KeSMSuSecRwStLegrestInOutPosDelta_Val/1 -> [PosDelta]
  [PosDelta] -> Subsystem6/4(Delta)
  LyLR2LLgrstInwdOtwdTrgtPosCalib_TrgtPosArray_read/1 -> [LyLCalib]
  LgrstOpen4sLR2LLgrstInwdOtwdTrgtPosCalib_TrgtPosArray_read/1 -> [LgrstOpenLCalib]
  [LgrstOpenLIsTargetPosZone] -> ?
  [LgrstCloseLIsTargetPosZone] -> Subsystem1/8(LgrstCloseLIsTargetPosZone)
  [VIPLIsTargetPosZone] -> Subsystem1/10(VIPLIsTargetPosZone)
  [PosDelta] -> Subsystem4/4(Delta)
  Subsystem5/2(IsPosZone) -> [RecvLIsTargetPosZone]
  [RecvLCalib] -> Subsystem/5(RecvLCalib)
  [RecvLIsTargetPosAlready] -> Subsystem1/6(RecvLIsTargetPosAlready)
  [RecvLCalib] -> Subsystem5/3(CalibArray)
  [LyLIsTargetPos] -> ?
  [LyLIsTargetPosAlready] -> ?
  [RecvLIsTargetPos] -> Subsystem1/3(RecvLIsTargetPos)
  Subsystem1/2(IsTargetPosAlready) -> Data Type Conversion2/1
  [LgrstCloseLIsTargetPosAlready] -> Subsystem1/5(LgrstCloseLIsTargetPosAlready)
  [PosDelta] -> Subsystem5/4(Delta)
  [VIPLIsTargetPos] -> Subsystem1/4(VIPLIsTargetPos)
  Subsystem5/1(IsPos) -> [RecvLIsTargetPos]
  Subsystem6/2(IsPosZone) -> [VIPLIsTargetPosZone]
  [LyLCalib] -> Subsystem4/3(CalibArray)
  [PosV] -> Subsystem2/1(PosV)
  IfVeSMSuSecRwLtStLgrstOtwdInwdPos_Val_read/1 -> [Pos]
  Data Type Conversion3/1 -> MdXXSecRwLtStLgrstInwdOtwdIsTargetPosZone_Val_write/1
  Subsystem5/3(IsPosAlready) -> [RecvLIsTargetPosAlready]
  [LyLCalib] -> Subsystem/4(LyLCalib)
  [PosV] -> Subsystem5/1(PosV)
  [PosV] -> Subsystem4/1(PosV)
  [LgrstCloseLIsTargetPos] -> Subsystem1/2(LgrstCloseLIsTargetPos)
  Subsystem/1(TrgtPos) -> Data Type Conversion/1
  [Pos] -> Subsystem6/2(Pos)
  Subsystem3/2(IsPosZone) -> [LgrstCloseLIsTargetPosZone]
  [RecvLIsTargetPosZone] -> Subsystem1/9(RecvLIsTargetPosZone)
  [Pos] -> Subsystem2/2(Pos)
  RecvLR2LLgrstInwdOtwdTrgtPosCalib_TrgtPosArray_read/1 -> [RecvLCalib]
  [Pos] -> Subsystem5/2(Pos)
  [LyLIsTargetPosZone] -> ?
  Subsystem3/1(IsPos) -> [LgrstCloseLIsTargetPos]
  Subsystem4/3(IsPosAlready) -> [LyLIsTargetPosAlready]
  [PosV] -> Subsystem3/1(PosV)
  [LgrstCloseLCalib] -> Subsystem/3(LgrstCloseLCalib)
  [MovConfig] -> Subsystem1/1(MovConfig)
  [PosTolr] -> Subsystem2/5(Tolr)
  Data Type Conversion/1 -> SecRwLtStLgrstInwdOtwdTrgtPos_Val_write/1
  [PosDelta] -> Subsystem2/4(Delta)
  Subsystem6/1(IsPos) -> [VIPLIsTargetPos]
  [Pos] -> Subsystem4/2(Pos)
  Subsystem3/3(IsPosAlready) -> [LgrstCloseLIsTargetPosAlready]
  Subsystem2/3(IsPosAlready) -> [LgrstOpenLIsTargetPosAlready]
  modestate32_Val_read/1 -> Subsystem/1(modestate32_Val_read)
  [PosV] -> Subsystem6/1(PosV)
  Subsystem6/3(IsPosAlready) -> [VIPLIsTargetPosAlready]
  Subsystem2/1(IsPos) -> [LgrstOpenLIsTargetPos]
  Subsystem4/1(IsPos) -> [LyLIsTargetPos]
  Data Type Conversion1/1 -> MdXXSecRwLtStLgrstInwdOtwdIsTargetPos_Val_write/1
  KeSMSw4SAcsMd22LgrstInwdOtwdTrgtPosCalib_TrgtPosArray_read/1 -> [Md22Calib]
  KeSMSw4SAcsMd26LgrstInwdOtwdTrgtPosCalib_TrgtPosArray_read/1 -> [Md26Calib]
  Subsystem7/3(IsPosAlready) -> [Md22IsTargetPosAlready]
  [PosV] -> Subsystem7/1(PosV)
  Subsystem7/1(IsPos) -> [Md22IsTargetPos]
  [Pos] -> Subsystem7/2(Pos)
  [Md22Calib] -> Subsystem7/3(CalibArray)
  Subsystem7/2(IsPosZone) -> [Md22IsTargetPosZone]
  [PosDelta] -> Subsystem7/4(Delta)
  [PosTolr] -> Subsystem7/5(Tolr)
  [PosTolr] -> Subsystem8/5(Tolr)
  [PosDelta] -> Subsystem8/4(Delta)
  Subsystem8/2(IsPosZone) -> [Md26IsTargetPosZone]
  [Md26Calib] -> Subsystem8/3(CalibArray)
  [Pos] -> Subsystem8/2(Pos)
  Subsystem8/1(IsPos) -> [Md26IsTargetPos]
  [PosV] -> Subsystem8/1(PosV)
  Subsystem8/3(IsPosAlready) -> [Md26IsTargetPosAlready]
  [Md26Calib] -> Subsystem/8(Md26Calib)
  [Md22Calib] -> Subsystem/7(Md22Calib)
  [Md22IsTargetPos] -> Subsystem1/11(Md22IsTargetPos)
  [Md26IsTargetPos] -> Subsystem1/12(Md26IsTargetPos)
  [Md22IsTargetPosAlready] -> Subsystem1/13(Md22IsTargetPosAlready)
  [Md26IsTargetPosAlready] -> Subsystem1/14(Md26IsTargetPosAlready)
  [Md22IsTargetPosZone] -> Subsystem1/15(Md22IsTargetPosZone)
  [Md26IsTargetPosZone] -> Subsystem1/16(Md26IsTargetPosZone)
  [LgrstCloseLCalib] -> Subsystem3/3(CalibArray)
  [LgrstOpenLCalib] -> Subsystem2/3(CalibArray)
  Subsystem9/3(IsPosAlready) -> [Md1IsTargetPosAlready]
  [PosV] -> Subsystem9/1(PosV)
  Subsystem9/1(IsPos) -> [Md1IsTargetPos]
  [Pos] -> Subsystem9/2(Pos)
  [Md1Calib] -> Subsystem9/3(CalibArray)
  Subsystem9/2(IsPosZone) -> [Md1IsTargetPosZone]
  [PosDelta] -> Subsystem9/4(Delta)
  [PosTolr] -> Subsystem9/5(Tolr)
  KeSMSwEZEEntryLgrstInwdOtwdTrgtPosCalib_TrgtPosArray_read/1 -> [Md1Calib]
  [Md1Calib] -> Subsystem/9(Md1Calib)
  [Md1IsTargetPos] -> Subsystem1/17(Md1IsTargetPos)
  [Md1IsTargetPosZone] -> Subsystem1/19(Md1IsTargetPosZone)
  [Md1IsTargetPosAlready] -> Subsystem1/18(Md1IsTargetPosAlready)
  VIPLExitR2LLgrstInwdOtwdTrgtPosCalib_TrgtPosArray_read/1 -> [Md27Calib]
  VIPLR2LLgrstInwdOtwdTrgtPosCalib_TrgtPosArray_read/1 -> [VIPL6s7sCalib]
  Switch/1 -> [VIPLCalib], Subsystem6/3(CalibArray)
  StNumFlg_Is6s7s_read/1 -> Switch/2
  Subsystem10/1(IsPos) -> [Md27IsTargetPos]
  [PosTolr] -> Subsystem10/5(Tolr)
  Subsystem10/2(IsPosZone) -> [Md27IsTargetPosZone]
  Subsystem10/3(IsPosAlready) -> [Md27IsTargetPosAlready]
  [PosV] -> Subsystem10/1(PosV)
  [Md27Calib] -> Subsystem10/3(CalibArray)
  [Pos] -> Subsystem10/2(Pos)
  [PosDelta] -> Subsystem10/4(Delta)
  [Md27Calib] -> Subsystem/10(Md27Calib)
  [Md27IsTargetPos] -> Subsystem1/20(Md27IsTargetPos)
  [Md27IsTargetPosAlready] -> Subsystem1/21(Md27IsTargetPosAlready)
  [Md27IsTargetPosZone] -> Subsystem1/22(Md27IsTargetPosZone)
  StNumFlg_Is7s_read/1 -> Subsystem1/23(StNumFlg_Is7s_read)
  Md8R2LLgrstInwdOtwdTrgtPosCalib_TrgtPosArray_read/1 -> [Md8Calib]
  Md56R2LLgrstInwdOtwdTrgtPosCalib_TrgtPosArray_read/1 -> [Md56Calib]
  [PosDelta] -> Subsystem11/4(Delta)
  [Pos] -> Subsystem11/2(Pos)
  [Md8Calib] -> Subsystem11/3(CalibArray)
  [PosV] -> Subsystem11/1(PosV)
  Subsystem11/3(IsPosAlready) -> [Md8IsTargetPosAlready]
  Subsystem11/2(IsPosZone) -> [Md8IsTargetPosZone]
  [PosTolr] -> Subsystem11/5(Tolr)
  Subsystem11/1(IsPos) -> [Md8IsTargetPos]
  Subsystem12/1(IsPos) -> [Md56IsTargetPos]
  [PosTolr] -> Subsystem12/5(Tolr)
  Subsystem12/2(IsPosZone) -> [Md56IsTargetPosZone]
  Subsystem12/3(IsPosAlready) -> [Md56IsTargetPosAlready]
  [PosV] -> Subsystem12/1(PosV)
  [Md56Calib] -> Subsystem12/3(CalibArray)
  [Pos] -> Subsystem12/2(Pos)
  [PosDelta] -> Subsystem12/4(Delta)
  [VIPL6s7sCalib] -> Switch/1
  [VIPL4sCalib] -> Switch/3
  [Md8Calib] -> Subsystem/11(Md8Calib)
  [Md56Calib] -> Subsystem/12(Md56Calib)
  [Md8IsTargetPos] -> Subsystem1/24(Md8IsTargetPos)
  [Md56IsTargetPos] -> Subsystem1/25(Md56IsTargetPos)
  [Md8IsTargetPosAlready] -> Subsystem1/26(Md8IsTargetPosAlready)
  [Md56IsTargetPosAlready] -> Subsystem1/27(Md56IsTargetPosAlready)
  [Md8IsTargetPosZone] -> Subsystem1/28(Md8IsTargetPosZone)
  [Md56IsTargetPosZone] -> Subsystem1/29(Md56IsTargetPosZone)
  Data Type Conversion2/1 -> Switch1/3, Bitwise Operator/1
  Switch1/1 -> MdXXSecRwLtStLgrstInwdOtwdIsTargetPosAlready_Val_write/1
  Constant/1 -> Bitwise Operator1/1
  Bitwise Operator/1 -> Switch1/1
  Bitwise Operator1/1 -> Bitwise Operator/2
  IfVeSMSbSecRwLtStCshnFrntUpwdDnwdMovConfig_Val_read/1 -> Switch1/2
  Md61SecRwLtStLgrstInwdOtwdTrgtPosCalib_TrgtPosArray_read/1 -> [Md61Calib]
  Md62SecRwLtStLgrstInwdOtwdTrgtPosCalib_TrgtPosArray_read/1 -> [Md62Calib]
  [PosDelta] -> Subsystem13/4(Delta)
  [Pos] -> Subsystem13/2(Pos)
  [Md61Calib] -> Subsystem13/3(CalibArray)
  [PosV] -> Subsystem13/1(PosV)
  Subsystem13/3(IsPosAlready) -> [Md61IsTargetPosAlready]
  Subsystem13/2(IsPosZone) -> [Md61IsTargetPosZone]
  [PosTolr] -> Subsystem13/5(Tolr)
  Subsystem13/1(IsPos) -> [Md61IsTargetPos]
  Subsystem14/1(IsPos) -> [Md62IsTargetPos]
  [PosTolr] -> Subsystem14/5(Tolr)
  Subsystem14/2(IsPosZone) -> [Md62IsTargetPosZone]
  Subsystem14/3(IsPosAlready) -> [Md62IsTargetPosAlready]
  [PosV] -> Subsystem14/1(PosV)
  [Md62Calib] -> Subsystem14/3(CalibArray)
  [Pos] -> Subsystem14/2(Pos)
  [PosDelta] -> Subsystem14/4(Delta)
  [Md62Calib] -> Subsystem/14(Md62Calib)
  [Md61Calib] -> Subsystem/13(Md61Calib)
  [Md61IsTargetPos] -> Subsystem1/30(Md61IsTargetPos)
  [Md62IsTargetPos] -> Subsystem1/31(Md62IsTargetPos)
  [Md62IsTargetPosZone] -> Subsystem1/35(Md62IsTargetPosZone)
  [Md61IsTargetPosZone] -> Subsystem1/34(Md61IsTargetPosZone)
  [Md62IsTargetPosAlready] -> Subsystem1/33(Md62IsTargetPosAlready)
  [Md61IsTargetPosAlready] -> Subsystem1/32(Md61IsTargetPosAlready)
  Relational Operator2/1 -> Logical Operator3/1
  Unit Delay3/1 -> Relational Operator3/2
  Unit Delay2/1 -> Relational Operator2/2
  Relational Operator3/1 -> Logical Operator3/2
  [Pos] -> Unit Delay3/1, Relational Operator3/1
  IfVeSMSuSecRwLtStLgrstUpwdDnwdPos_Val_read/1 -> Unit Delay2/1, Relational Operator2/1
  Logical Operator3/1 -> SecRwLtStLgrstInwdOtwdNotMovFlg_Val_write/1

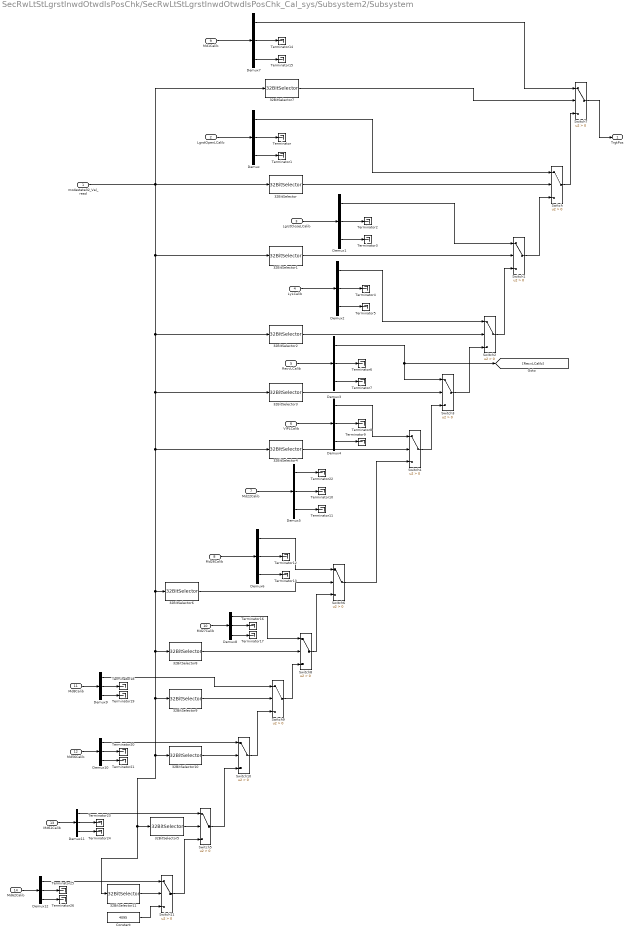
== system SecRwLtStLgrstInwdOtwdIsPosChk/SecRwLtStLgrstInwdOtwdIsPosChk_Cal_sys/Subsystem2/Subsystem ==
  modestate32_Val_read : Inport
  LgrstOpenLCalib : Inport  Port=2
  LgrstCloseLCalib : Inport  Port=3
  LyLCalib : Inport  Port=4
  RecvLCalib : Inport  Port=5
  VIPLCalib : Inport  Port=6
  Md22Calib : Inport  Port=7
  Md26Calib : Inport  Port=8
  Md1Calib : Inport  Port=9
  Md27Calib : Inport  Port=10
  Md8Calib : Inport  Port=11
  Md56Calib : Inport  Port=12
  Md61Calib : Inport  Port=13
  Md62Calib : Inport  Port=14
  32BitSelector : StIsPosChkLib/32BitSelector  BitNum=15
  32BitSelector1 : StIsPosChkLib/32BitSelector  BitNum=16
  32BitSelector10 : StIsPosChkLib/32BitSelector  BitNum=24
  32BitSelector11 : StIsPosChkLib/32BitSelector  BitNum=6
  32BitSelector2 : StIsPosChkLib/32BitSelector  BitNum=13
  32BitSelector3 : StIsPosChkLib/32BitSelector  BitNum=10
  32BitSelector4 : StIsPosChkLib/32BitSelector  BitNum=9
  32BitSelector5 : StIsPosChkLib/32BitSelector  BitNum=5
  32BitSelector6 : StIsPosChkLib/32BitSelector  BitNum=25
  32BitSelector7 : StIsPosChkLib/32BitSelector  BitNum=0
  32BitSelector8 : StIsPosChkLib/32BitSelector  BitNum=26
  32BitSelector9 : StIsPosChkLib/32BitSelector  BitNum=7
  Constant : Constant  Value=4095  OutDataTypeStr=uint16
  Demux{,1..12} (13 alike) : Demux  Outputs=3
  Switch{,1..11} (12 alike) : Switch  Criteria=u2 > Threshold  SaturateOnIntegerOverflow=off  InputSameDT=off
  Terminator{,1..26} (27 alike) : Terminator
  TrgtPos : Outport  VectorParamsAs1DForOutWhenUnconnected=off
      settings: EnsureOutportIsVirtual=on
  wires:
  32BitSelector/1 -> Switch/2
  Demux/1 -> Switch/1
  Demux/3 -> Terminator1/1
  Demux/2 -> Terminator/1
  LgrstOpenLCalib/1 -> Demux/1
  LgrstCloseLCalib/1 -> Demux1/1
  Demux1/2 -> Terminator2/1
  Demux1/3 -> Terminator3/1
  Demux1/1 -> Switch1/1
  Switch1/1 -> Switch/3
  32BitSelector1/1 -> Switch1/2
  Switch2/1 -> Switch1/3
  Switch3/1 -> Switch2/3
  Switch4/1 -> Switch3/3
  32BitSelector2/1 -> Switch2/2
  32BitSelector3/1 -> Switch3/2
  32BitSelector4/1 -> Switch4/2
  Demux2/1 -> Switch2/1
  Demux2/3 -> Terminator5/1
  Demux2/2 -> Terminator4/1
  LyLCalib/1 -> Demux2/1
  RecvLCalib/1 -> Demux3/1
  Demux3/2 -> Terminator6/1
  Demux3/3 -> Terminator7/1
  Demux3/1 -> Switch3/1, [RecvLCalib]
  Demux4/1 -> Switch4/1
  Demux4/3 -> Terminator9/1
  Demux4/2 -> Terminator8/1
  VIPLCalib/1 -> Demux4/1
  Md22Calib/1 -> Demux5/1
  Demux5/2 -> Terminator10/1
  Demux5/3 -> Terminator11/1
  Demux5/1 -> Terminator22/1
  modestate32_Val_read/1 -> 32BitSelector7/1, 32BitSelector/1, 32BitSelector1/1, 32BitSelector2/1, 32BitSelector3/1, 32BitSelector11/1, 32BitSelector5/1, 32BitSelector10/1, 32BitSelector9/1, 32BitSelector8/1, 32BitSelector6/1, 32BitSelector4/1
  32BitSelector6/1 -> Switch6/2
  Demux6/1 -> Switch6/1
  Demux6/3 -> Terminator13/1
  Demux6/2 -> Terminator12/1
  Md26Calib/1 -> Demux6/1
  Switch6/1 -> Switch4/3
  Switch7/1 -> TrgtPos/1
  Switch/1 -> Switch7/3
  32BitSelector7/1 -> Switch7/2
  Md1Calib/1 -> Demux7/1
  Demux7/2 -> Terminator14/1
  Demux7/3 -> Terminator15/1
  Demux7/1 -> Switch7/1
  Demux8/2 -> Terminator16/1
  Demux8/3 -> Terminator17/1
  Md27Calib/1 -> Demux8/1
  Demux8/1 -> Switch8/1
  Switch8/1 -> Switch6/3
  32BitSelector8/1 -> Switch8/2
  Switch9/1 -> Switch8/3
  32BitSelector9/1 -> Switch9/2
  Demux9/1 -> Switch9/1
  Md8Calib/1 -> Demux9/1
  Demux9/3 -> Terminator19/1
  Demux9/2 -> Terminator18/1
  Demux10/2 -> Terminator20/1
  Demux10/3 -> Terminator21/1
  Md56Calib/1 -> Demux10/1
  Demux10/1 -> Switch10/1
  Switch10/1 -> Switch9/3
  32BitSelector10/1 -> Switch10/2
  Switch5/1 -> Switch10/3
  Switch11/1 -> Switch5/3
  32BitSelector11/1 -> Switch11/2
  32BitSelector5/1 -> Switch5/2
  Constant/1 -> Switch11/3
  Demux11/1 -> Switch5/1
  Md61Calib/1 -> Demux11/1
  Demux11/3 -> Terminator24/1
  Demux11/2 -> Terminator23/1
  Demux12/2 -> Terminator25/1
  Demux12/3 -> Terminator26/1
  Md62Calib/1 -> Demux12/1
  Demux12/1 -> Switch11/1

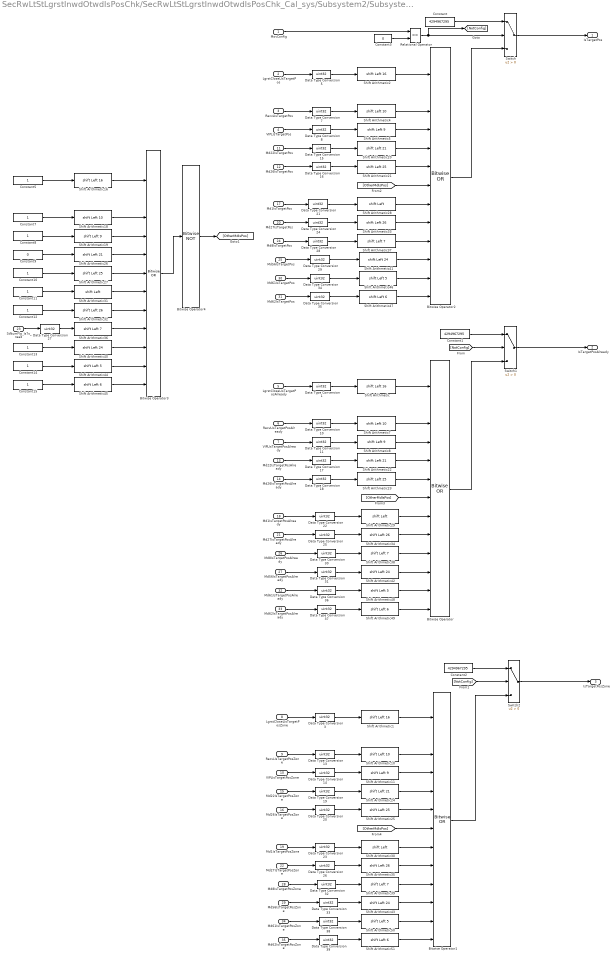
== system SecRwLtStLgrstInwdOtwdIsPosChk/SecRwLtStLgrstInwdOtwdIsPosChk_Cal_sys/Subsystem2/Subsystem1 ==
  MovConfig : Inport
  LgrstCloseLIsTargetPos : Inport  Port=2
  RecvLIsTargetPos : Inport  Port=3
  VIPLIsTargetPos : Inport  Port=4
  LgrstCloseLIsTargetPosAlready : Inport  Port=5
  RecvLIsTargetPosAlready : Inport  Port=6
  VIPLIsTargetPosAlready : Inport  Port=7
  LgrstCloseLIsTargetPosZone : Inport  Port=8
  RecvLIsTargetPosZone : Inport  Port=9
  VIPLIsTargetPosZone : Inport  Port=10
  Md22IsTargetPos : Inport  Port=11
  Md26IsTargetPos : Inport  Port=12
  Md22IsTargetPosAlready : Inport  Port=13
  Md26IsTargetPosAlready : Inport  Port=14
  Md22IsTargetPosZone : Inport  Port=15
  Md26IsTargetPosZone : Inport  Port=16
  Md1IsTargetPos : Inport  Port=17
  Md1IsTargetPosAlready : Inport  Port=18
  Md1IsTargetPosZone : Inport  Port=19
  Md27IsTargetPos : Inport  Port=20
  Md27IsTargetPosAlready : Inport  Port=21
  Md27IsTargetPosZone : Inport  Port=22
  StNumFlg_Is7s_read : Inport  Port=23
  Md8IsTargetPos : Inport  Port=24
  Md56IsTargetPos : Inport  Port=25
  Md8IsTargetPosAlready : Inport  Port=26
  Md56IsTargetPosAlready : Inport  Port=27
  Md8IsTargetPosZone : Inport  Port=28
  Md56IsTargetPosZone : Inport  Port=29
  Md61IsTargetPos : Inport  Port=30
  Md62IsTargetPos : Inport  Port=31
  Md61IsTargetPosAlready : Inport  Port=32
  Md62IsTargetPosAlready : Inport  Port=33
  Md61IsTargetPosZone : Inport  Port=34
  Md62IsTargetPosZone : Inport  Port=35
  Bitwise Operator : simulink/Logic and Bit Operations/Bitwise Operator  logicop=OR  UseBitMask=off  NumInputPorts=14  BitMask=bin2dec('11011001')  BitMaskRealWorld=Stored Integer
  Bitwise Operator1 : simulink/Logic and Bit Operations/Bitwise Operator  logicop=OR  UseBitMask=off  NumInputPorts=14  BitMask=bin2dec('11011001')  BitMaskRealWorld=Stored Integer
  Bitwise Operator2 : simulink/Logic and Bit Operations/Bitwise Operator  logicop=OR  UseBitMask=off  NumInputPorts=14  BitMask=bin2dec('11011001')  BitMaskRealWorld=Stored Integer
  Bitwise Operator3 : simulink/Logic and Bit Operations/Bitwise Operator  logicop=OR  UseBitMask=off  NumInputPorts=13  BitMask=bin2dec('11011001')  BitMaskRealWorld=Stored Integer
  Bitwise Operator4 : simulink/Logic and Bit Operations/Bitwise Operator  logicop=NOT  UseBitMask=off  BitMask=bin2dec('11011001')  BitMaskRealWorld=Stored Integer
  Constant : Constant  Value=4294967295  OutDataTypeStr=uint32
  Constant1 : Constant  Value=4294967295  OutDataTypeStr=uint32
  Constant{5,7..8,10..15} (9 alike) : Constant  OutDataTypeStr=uint32
  Constant2 : Constant  Value=4294967295  OutDataTypeStr=uint32
  Constant3 : Constant  Value=0  OutDataTypeStr=uint8
  Constant9 : Constant  Value=0  OutDataTypeStr=uint32
  Data Type Conversion{1,3,5,7..8,10..11,13..39} (34 alike) : DataTypeConversion  OutDataTypeStr=uint32  SaturateOnIntegerOverflow=off  RndMeth=Floor
  Relational Operator : RelationalOperator  Operator===  OutDataTypeStr=boolean  RndMeth=Simplest  InputSameDT=off
  Shift Arithmetic{,1..2,16} (4 alike) : ArithShift  BitShiftNumber=16  BitShiftDirection=Left
  Shift Arithmetic{4,7,10,18} (4 alike) : ArithShift  BitShiftNumber=10  BitShiftDirection=Left
  Shift Arithmetic{5,8,11,19} (4 alike) : ArithShift  BitShiftNumber=9  BitShiftDirection=Left
  Shift Arithmetic{20,22,24,26} (4 alike) : ArithShift  BitShiftNumber=21  BitShiftDirection=Left
  Shift Arithmetic{21,23,25,27} (4 alike) : ArithShift  BitShiftNumber=25  BitShiftDirection=Left
  Shift Arithmetic{28..31} (4 alike) : ArithShift  BitShiftDirection=Left
  Shift Arithmetic{32..35} (4 alike) : ArithShift  BitShiftNumber=26  BitShiftDirection=Left
  Shift Arithmetic{36..39} (4 alike) : ArithShift  BitShiftNumber=7  BitShiftDirection=Left
  Shift Arithmetic{40..43} (4 alike) : ArithShift  BitShiftNumber=24  BitShiftDirection=Left
  Shift Arithmetic{44,46,48,50} (4 alike) : ArithShift  BitShiftNumber=5  BitShiftDirection=Left
  Shift Arithmetic{45,47,49,51} (4 alike) : ArithShift  BitShiftNumber=6  BitShiftDirection=Left
  Switch : Switch  Criteria=u2 > Threshold  SaturateOnIntegerOverflow=off  InputSameDT=off
  Switch1 : Switch  Criteria=u2 > Threshold  SaturateOnIntegerOverflow=off  InputSameDT=off
  Switch2 : Switch  Criteria=u2 > Threshold  SaturateOnIntegerOverflow=off  InputSameDT=off
  IsTargetPos : Outport  VectorParamsAs1DForOutWhenUnconnected=off
      settings: EnsureOutportIsVirtual=on
  IsTargetPosAlready : Outport  Port=2  VectorParamsAs1DForOutWhenUnconnected=off
      settings: EnsureOutportIsVirtual=on
  IsTargetPosZone : Outport  Port=3  VectorParamsAs1DForOutWhenUnconnected=off
      settings: EnsureOutportIsVirtual=on
  wires:
  Constant3/1 -> Relational Operator/2
  Constant/1 -> Switch/1
  Relational Operator/1 -> [NotConfig], Switch/2
  MovConfig/1 -> Relational Operator/1
  Switch/1 -> IsTargetPos/1
  [NotConfig] -> Switch1/2
  Constant1/1 -> Switch1/1
  Switch1/1 -> IsTargetPosAlready/1
  Switch2/1 -> IsTargetPosZone/1
  Constant2/1 -> Switch2/1
  [NotConfig] -> Switch2/2
  Data Type Conversion1/1 -> Shift Arithmetic/1
  Shift Arithmetic/1 -> Bitwise Operator/2
  Shift Arithmetic1/1 -> Bitwise Operator1/2
  Data Type Conversion3/1 -> Shift Arithmetic1/1
  Bitwise Operator1/1 -> Switch2/3
  Bitwise Operator/1 -> Switch1/3
  Shift Arithmetic2/1 -> Bitwise Operator2/2
  Data Type Conversion5/1 -> Shift Arithmetic2/1
  Bitwise Operator2/1 -> Switch/3
  LgrstCloseLIsTargetPos/1 -> Data Type Conversion5/1
  LgrstCloseLIsTargetPosZone/1 -> Data Type Conversion3/1
  LgrstCloseLIsTargetPosAlready/1 -> Data Type Conversion1/1
  Shift Arithmetic4/1 -> Bitwise Operator2/4
  Shift Arithmetic5/1 -> Bitwise Operator2/5
  Data Type Conversion7/1 -> Shift Arithmetic4/1
  Data Type Conversion8/1 -> Shift Arithmetic5/1
  RecvLIsTargetPos/1 -> Data Type Conversion7/1
  VIPLIsTargetPos/1 -> Data Type Conversion8/1
  VIPLIsTargetPosAlready/1 -> Data Type Conversion11/1
  RecvLIsTargetPosAlready/1 -> Data Type Conversion10/1
  Data Type Conversion11/1 -> Shift Arithmetic8/1
  Data Type Conversion10/1 -> Shift Arithmetic7/1
  Shift Arithmetic8/1 -> Bitwise Operator/5
  Shift Arithmetic7/1 -> Bitwise Operator/4
  Data Type Conversion14/1 -> Shift Arithmetic11/1
  Data Type Conversion13/1 -> Shift Arithmetic10/1
  VIPLIsTargetPosZone/1 -> Data Type Conversion14/1
  Shift Arithmetic10/1 -> Bitwise Operator1/4
  RecvLIsTargetPosZone/1 -> Data Type Conversion13/1
  Shift Arithmetic11/1 -> Bitwise Operator1/5
  Shift Arithmetic19/1 -> Bitwise Operator3/5
  Shift Arithmetic18/1 -> Bitwise Operator3/4
  Shift Arithmetic16/1 -> Bitwise Operator3/2
  Constant5/1 -> Shift Arithmetic16/1
  Constant7/1 -> Shift Arithmetic18/1
  Constant8/1 -> Shift Arithmetic19/1
  Bitwise Operator3/1 -> Bitwise Operator4/1
  Bitwise Operator4/1 -> [OtherMdIsPos]
  [OtherMdIsPos] -> Bitwise Operator2/8
  Md22IsTargetPos/1 -> Data Type Conversion15/1
  Data Type Conversion15/1 -> Shift Arithmetic20/1
  Shift Arithmetic20/1 -> Bitwise Operator2/6
  Shift Arithmetic21/1 -> Bitwise Operator2/7
  Data Type Conversion16/1 -> Shift Arithmetic21/1
  Md26IsTargetPos/1 -> Data Type Conversion16/1
  [OtherMdIsPos] -> Bitwise Operator/8
  Shift Arithmetic22/1 -> Bitwise Operator/6
  Data Type Conversion17/1 -> Shift Arithmetic22/1
  Md22IsTargetPosAlready/1 -> Data Type Conversion17/1
  Md26IsTargetPosAlready/1 -> Data Type Conversion18/1
  Data Type Conversion18/1 -> Shift Arithmetic23/1
  Shift Arithmetic23/1 -> Bitwise Operator/7
  [OtherMdIsPos] -> Bitwise Operator1/8
  Shift Arithmetic24/1 -> Bitwise Operator1/6
  Md22IsTargetPosZone/1 -> Data Type Conversion19/1
  Data Type Conversion19/1 -> Shift Arithmetic24/1
  Data Type Conversion20/1 -> Shift Arithmetic25/1
  Md26IsTargetPosZone/1 -> Data Type Conversion20/1
  Shift Arithmetic25/1 -> Bitwise Operator1/7
  Constant9/1 -> Shift Arithmetic26/1
  Shift Arithmetic26/1 -> Bitwise Operator3/6
  Shift Arithmetic27/1 -> Bitwise Operator3/7
  Constant10/1 -> Shift Arithmetic27/1
  Md1IsTargetPosZone/1 -> Data Type Conversion23/1
  Md1IsTargetPosAlready/1 -> Data Type Conversion22/1
  Md1IsTargetPos/1 -> Data Type Conversion21/1
  Data Type Conversion21/1 -> Shift Arithmetic28/1
  Shift Arithmetic28/1 -> Bitwise Operator2/9
  Shift Arithmetic29/1 -> Bitwise Operator/9
  Data Type Conversion22/1 -> Shift Arithmetic29/1
  Shift Arithmetic30/1 -> Bitwise Operator1/9
  Data Type Conversion23/1 -> Shift Arithmetic30/1
  Constant11/1 -> Shift Arithmetic31/1
  Shift Arithmetic31/1 -> Bitwise Operator3/8
  Shift Arithmetic32/1 -> Bitwise Operator3/9
  Constant12/1 -> Shift Arithmetic32/1
  Shift Arithmetic33/1 -> Bitwise Operator2/10
  Data Type Conversion24/1 -> Shift Arithmetic33/1
  Md27IsTargetPos/1 -> Data Type Conversion24/1
  Data Type Conversion25/1 -> Shift Arithmetic34/1
  Shift Arithmetic34/1 -> Bitwise Operator/10
  Md27IsTargetPosAlready/1 -> Data Type Conversion25/1
  Data Type Conversion26/1 -> Shift Arithmetic35/1
  Shift Arithmetic35/1 -> Bitwise Operator1/10
  Md27IsTargetPosZone/1 -> Data Type Conversion26/1
  StNumFlg_Is7s_read/1 -> Data Type Conversion27/1
  Shift Arithmetic36/1 -> Bitwise Operator3/10
  Shift Arithmetic37/1 -> Bitwise Operator2/11
  Shift Arithmetic38/1 -> Bitwise Operator/11
  Shift Arithmetic39/1 -> Bitwise Operator1/11
  Data Type Conversion27/1 -> Shift Arithmetic36/1
  Constant13/1 -> Shift Arithmetic40/1
  Shift Arithmetic40/1 -> Bitwise Operator3/11
  Md8IsTargetPos/1 -> Data Type Conversion28/1
  Data Type Conversion28/1 -> Shift Arithmetic37/1
  Data Type Conversion29/1 -> Shift Arithmetic41/1
  Md56IsTargetPos/1 -> Data Type Conversion29/1
  Shift Arithmetic41/1 -> Bitwise Operator2/12
  Md8IsTargetPosAlready/1 -> Data Type Conversion30/1
  Data Type Conversion30/1 -> Shift Arithmetic38/1
  Data Type Conversion31/1 -> Shift Arithmetic42/1
  Md56IsTargetPosAlready/1 -> Data Type Conversion31/1
  Shift Arithmetic42/1 -> Bitwise Operator/12
  Md8IsTargetPosZone/1 -> Data Type Conversion32/1
  Data Type Conversion32/1 -> Shift Arithmetic39/1
  Data Type Conversion33/1 -> Shift Arithmetic43/1
  Md56IsTargetPosZone/1 -> Data Type Conversion33/1
  Shift Arithmetic43/1 -> Bitwise Operator1/12
  Shift Arithmetic44/1 -> Bitwise Operator3/12
  Constant14/1 -> Shift Arithmetic44/1
  Constant15/1 -> Shift Arithmetic45/1
  Shift Arithmetic45/1 -> Bitwise Operator3/13
  Shift Arithmetic46/1 -> Bitwise Operator2/13
  Md61IsTargetPos/1 -> Data Type Conversion34/1
  Data Type Conversion34/1 -> Shift Arithmetic46/1
  Data Type Conversion35/1 -> Shift Arithmetic47/1
  Md62IsTargetPos/1 -> Data Type Conversion35/1
  Shift Arithmetic47/1 -> Bitwise Operator2/14
  Shift Arithmetic48/1 -> Bitwise Operator/13
  Md61IsTargetPosAlready/1 -> Data Type Conversion36/1
  Data Type Conversion36/1 -> Shift Arithmetic48/1
  Data Type Conversion37/1 -> Shift Arithmetic49/1
  Md62IsTargetPosAlready/1 -> Data Type Conversion37/1
  Shift Arithmetic49/1 -> Bitwise Operator/14
  Shift Arithmetic50/1 -> Bitwise Operator1/13
  Md61IsTargetPosZone/1 -> Data Type Conversion38/1
  Data Type Conversion38/1 -> Shift Arithmetic50/1
  Data Type Conversion39/1 -> Shift Arithmetic51/1
  Md62IsTargetPosZone/1 -> Data Type Conversion39/1
  Shift Arithmetic51/1 -> Bitwise Operator1/14

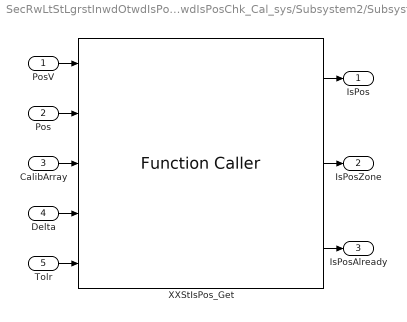
== system SecRwLtStLgrstInwdOtwdIsPosChk/SecRwLtStLgrstInwdOtwdIsPosChk_Cal_sys/Subsystem2/Subsystem10 ==
  PosV : Inport
  Pos : Inport  Port=2
  CalibArray : Inport  Port=3
  Delta : Inport  Port=4
  Tolr : Inport  Port=5
  XXStIsPos_Get : FunctionCaller  FunctionPrototype=[IsPos,IsPosZone,IsPosAlready] = XXStIsPos_Get(PosV,Pos,CalibArray,Delta,Tolr)  InputArgumentSpecifications=boolean(true), uint16(1), uint16([1;1;1]), uint16(1), uint16(1)  OutputArgumentSpecifications=boolean(true), boolean(true), boolean(true)
  IsPos : Outport  VectorParamsAs1DForOutWhenUnconnected=off
  IsPosZone : Outport  Port=2  VectorParamsAs1DForOutWhenUnconnected=off
  IsPosAlready : Outport  Port=3  VectorParamsAs1DForOutWhenUnconnected=off
  wires:
  PosV/1 -> XXStIsPos_Get/1
  Pos/1 -> XXStIsPos_Get/2
  XXStIsPos_Get/3 -> IsPosAlready/1
  Tolr/1 -> XXStIsPos_Get/5
  XXStIsPos_Get/1 -> IsPos/1
  XXStIsPos_Get/2 -> IsPosZone/1
  Delta/1 -> XXStIsPos_Get/4
  CalibArray/1 -> XXStIsPos_Get/3

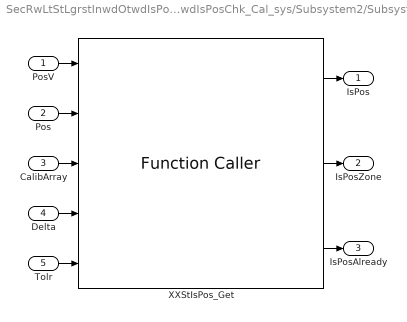
== system SecRwLtStLgrstInwdOtwdIsPosChk/SecRwLtStLgrstInwdOtwdIsPosChk_Cal_sys/Subsystem2/Subsystem11 ==
  PosV : Inport
  Pos : Inport  Port=2
  CalibArray : Inport  Port=3
  Delta : Inport  Port=4
  Tolr : Inport  Port=5
  XXStIsPos_Get : FunctionCaller  FunctionPrototype=[IsPos,IsPosZone,IsPosAlready] = XXStIsPos_Get(PosV,Pos,CalibArray,Delta,Tolr)  InputArgumentSpecifications=boolean(true), uint16(1), uint16([1;1;1]), uint16(1), uint16(1)  OutputArgumentSpecifications=boolean(true), boolean(true), boolean(true)
  IsPos : Outport  VectorParamsAs1DForOutWhenUnconnected=off
  IsPosZone : Outport  Port=2  VectorParamsAs1DForOutWhenUnconnected=off
  IsPosAlready : Outport  Port=3  VectorParamsAs1DForOutWhenUnconnected=off
  wires:
  CalibArray/1 -> XXStIsPos_Get/3
  Delta/1 -> XXStIsPos_Get/4
  XXStIsPos_Get/2 -> IsPosZone/1
  XXStIsPos_Get/1 -> IsPos/1
  Tolr/1 -> XXStIsPos_Get/5
  XXStIsPos_Get/3 -> IsPosAlready/1
  Pos/1 -> XXStIsPos_Get/2
  PosV/1 -> XXStIsPos_Get/1
